simulink model "PI_Deadzone"  (R2025b)
settings: Solver=VariableStepAuto  StartTime=0.0  StopTime=10.0  RelTol=1e-3
libraries: simulink x1
settings Model: Creator=Ilya  LastModifiedBy=Admin

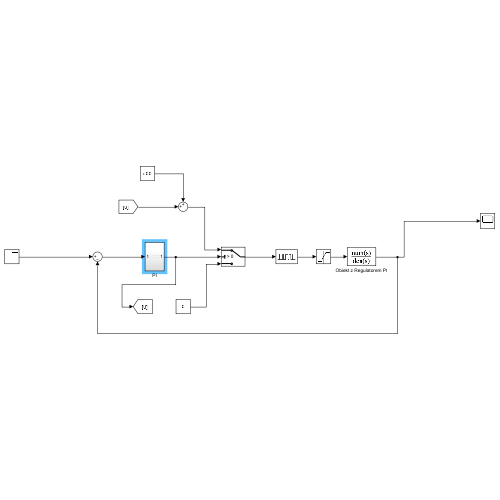
[thumbnail: Simulink's stored preview of the top-level diagram]
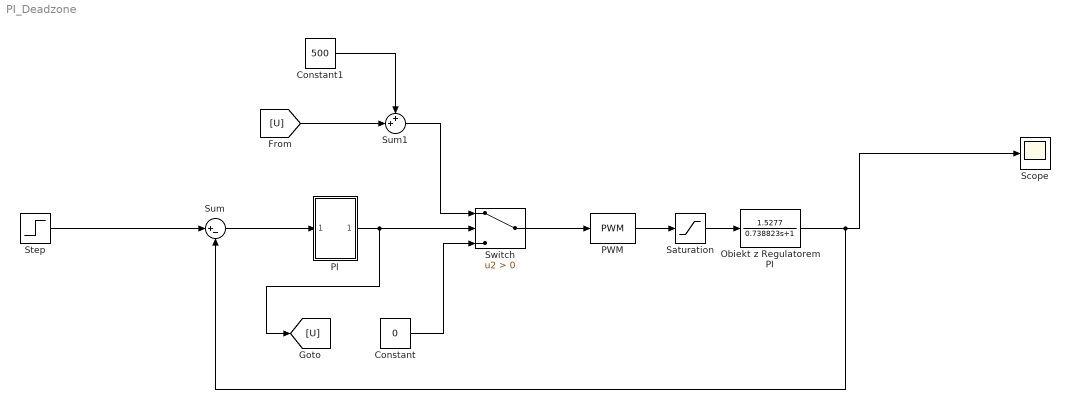
== system PI_Deadzone ==
  Constant : Constant  Value=0
  Constant1 : Constant  Value=500
  Obiekt z Regulatorem PI : TransferFcn  Numerator=[1.5277]  Denominator=[0.738823 1]
  PI : Subsystem
  PWM : simulink/Discontinuities/PWM  DisableCoverage=on  Period=0.01  InitialDelay=0  DisallowZeroDutyCycle=off  RunAtFixedTimeIntervals=off  SampleTime=0.1
  Saturation : Saturate  UpperLimit=1000  LowerLimit=0
  Scope : Scope
      settings: ActiveDisplayYMinimum=-0.19096  ActiveDisplayYMaximum=1.71866
  Step : Step  Time=0  After=80  SampleTime=0
  Sum : Sum  Inputs=|+-
  Sum1 : Sum  Inputs=++|
  Switch : Switch  Criteria=u2 > Threshold  SaturateOnIntegerOverflow=off  InputSameDT=off
  wires:
  Step/1 -> Sum/1
  Obiekt z Regulatorem PI/1 -> Scope/1, Sum/2
  Saturation/1 -> Obiekt z Regulatorem PI/1
  Sum/1 -> PI/1(In1)
  PI/1(Out1) -> Switch/2, [U]
  PWM/1 -> Saturation/1
  Switch/1 -> PWM/1
  Constant/1 -> Switch/3
  [U] -> Sum1/2
  Constant1/1 -> Sum1/1
  Sum1/1 -> Switch/1

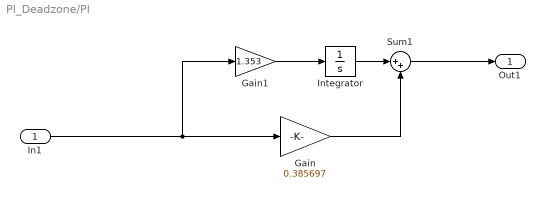
== system PI_Deadzone/PI ==
  In1 : Inport
  Gain : Gain  Gain=0.385697
  Gain1 : Gain  Gain=1.353
  Integrator : Integrator
  Sum1 : Sum  Inputs=|++
  Out1 : Outport
  wires:
  Gain1/1 -> Integrator/1
  In1/1 -> Gain1/1, Gain/1
  Integrator/1 -> Sum1/1
  Sum1/1 -> Out1/1
  Gain/1 -> Sum1/2
